simulink model "simF162"  (R2014a)
settings: Solver=ode45  StartTime=0.0  StopTime=20  RelTol=1e-3
values from neighbouring files (symbols this model uses):
  A = f16ss.a    [h2F16.m]    (also in h2F16ex2.m; h2F16ex3.m; h2F16ex_iconnect.m; h2cart.m = [0 0 1 0)
  B = [Bd Bu]    [h2F16.m]    (also in h2F16ex2.m = [Bu Bd]; h2F16ex3.m; h2F16ex_iconnect.m; hinfF16.m = [Bu Bd])
  Br = diag([100,1, 1, 1])    [h2F16.m]    (also in h2F16ex2.m = GAM - h2K*PI; h2F16ex3.m = S.b)
  Cy = [1  0 0 0 ... (first row only)    [h2F16ex2.m]    (also in h2F16ex3.m; h2F16ex_iconnect.m; hinfF16.m; hinfF16_v2.m = [0 -1 1 0])
  Gstep = 45*d2r    (= 0.785398163397)    [h2F16ex2.m]
  h2K = Z*inv(X)    [h2F16.m]    (also in h2F16ex2.m; h2F16ex3.m; h2cart.m; h2ex1.m)
  nd = 1    [h2F16.m]    (also in h2F16ex2.m; h2F16ex3.m; h2F16ex_iconnect.m)
  nu = 2    [h2F16.m]    (also in h2F16ex2.m; h2F16ex3.m; h2F16ex_iconnect.m; h2cart.m = 1)
  nx = 4    [h2F16.m]    (also in h2F16ex2.m; h2F16ex3.m; h2F16ex_iconnect.m; h2cart.m)
  Vstep = 50    [h2F16ex2.m]
  wd = 1    [h2F16.m]    (also in h2F16ex2.m; h2F16ex3.m; hinfF16.m; hinfF16_v2.m)
settings Model: Creator=raktim  LastModifiedBy=raktim

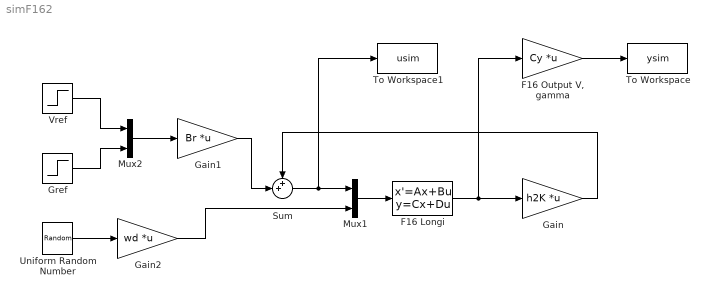
== system simF162 ==
  F16 Longi : StateSpace  A=A  B=B  C=eye(nx)  D=zeros(nx,nd+nu)  X0=0
  "F16 Output V, gamma" : Gain  Gain=Cy  Multiplication=Matrix(K*u)
  Gain : Gain  Gain=h2K  Multiplication=Matrix(K*u)
  Gain1 : Gain  Gain=Br  Multiplication=Matrix(K*u)
  Gain2 : Gain  Gain=wd  Multiplication=Matrix(K*u)
  Gref : Step  After=Gstep  SampleTime=0
  Mux1 : Mux  Inputs=2
  Mux2 : Mux  Inputs=2
  Sum : Sum  Inputs=++|
  To Workspace : ToWorkspace  VariableName=ysim  SaveFormat=Timeseries  SampleTime=-1
  To Workspace1 : ToWorkspace  VariableName=usim  SaveFormat=Timeseries  SampleTime=-1
  Uniform Random Number : UniformRandomNumber  SampleTime=0.01
  Vref : Step  Time=0  After=Vstep  SampleTime=0
  wires:
  F16 Longi/1 -> Gain/1, "F16 Output V, gamma"/1
  Gref/1 -> Mux2/2
  Vref/1 -> Mux2/1
  Mux2/1 -> Gain1/1
  Gain/1 -> Sum/1
  Gain1/1 -> Sum/2
  Sum/1 -> To Workspace1/1, Mux1/1
  Mux1/1 -> F16 Longi/1
  "F16 Output V, gamma"/1 -> To Workspace/1
  Uniform Random Number/1 -> Gain2/1
  Gain2/1 -> Mux1/2
